simulink model "Testing"  (R2023b)
settings: Solver=VariableStepAuto  StartTime=0.0  StopTime=10.0  RelTol=1e-3
settings Model: Creator=elija  LastModifiedBy=elija

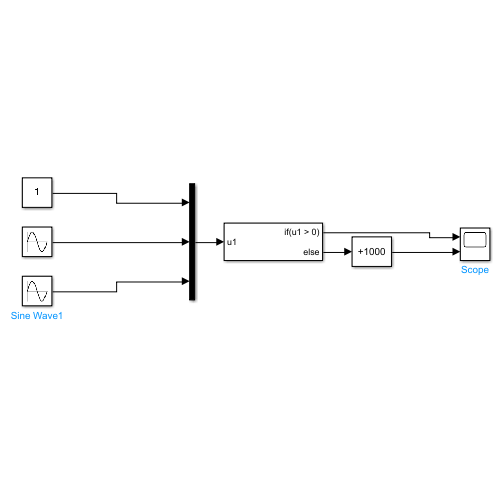
[thumbnail: Simulink's stored preview of the top-level diagram]
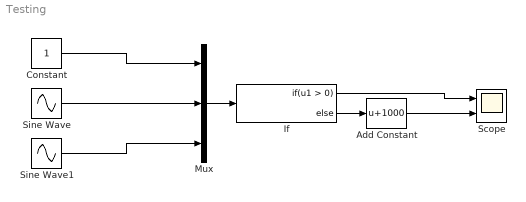
== system Testing ==
  Add Constant : Bias  Bias=1000  SaturateOnIntegerOverflow=off
  Constant : Constant
  If : If
  Mux : Mux  Inputs=3
  Scope : Scope  NumInputPorts=2
  Sine Wave : Sin  Amplitude=10  SampleTime=0
  Sine Wave1 : Sin  SampleTime=0
  wires:
  Sine Wave/1 -> Mux/2
  Constant/1 -> Mux/1
  Sine Wave1/1 -> Mux/3
  Mux/1 -> If/1
  If/2 -> Add Constant/1
  If/1 -> Scope/1
  Add Constant/1 -> Scope/2
